simulink model "MSE491_Lab2_sample"  (R2018a)
settings: Solver=ode4  StartTime=0.0  StopTime=1  FixedStep=0.0002  MaxStep=1e-4  RelTol=1e-3  EnableMultiTasking=on
settings Model: Creator=jw  LastModifiedBy=jw
settings DataIOCC: LimitDataPoints=on  SaveFormat=Array  SignalLoggingSaveFormat=ModelDataLogs
settings OptimizationCC: InitFltsAndDblsToZero=on  LifeSpan=inf
settings DebuggingCC: SaveWithParameterizedLinksMsg=none  UnderspecifiedInitializationDetection=Classic  MergeDetectMultiDrivingBlocksExec=none  SignalResolutionControl=TryResolveAllWithWarning  SolverPrmCheckMsg=warning  MultiTaskDSMMsg=warning  MultiTaskCondExecSysMsg=none  FcnCallInpInsideContextMsg=warning  SFUnexpectedBacktrackingDiag=warning  SFNoUnconditionalDefaultTransitionDiag=warning  SFExecutionAtInitializationDiag=none
settings HardwareCC: ProdBitPerPointer=32  ProdBitPerSizeT=32  ProdBitPerPtrDiffT=32  ProdLargestAtomicFloat=None  ProdIntDivRoundTo=Undefined  ProdEndianess=Unspecified  ProdWordSize=32  ProdHWDeviceType=32-bit Generic
settings ModelReferenceCC: PropagateSignalLabelsOutOfModel=off
settings CodeAppCC: StateflowObjectComments=on
settings GRTTargetCC: TargetFcnLib=ansi_tfl_tmw.mat  TargetLangStandard=C89/C90 (ANSI)  CombineOutputUpdateFcns=off  GRTInterface=on
settings ConfigComp: CovMetricSettings=dw  CovHtmlReporting=on  CovSaveCumulativeToWorkspaceVar=on  CovSaveSingleToWorkspaceVar=on  CovExternalEMLEnable=off

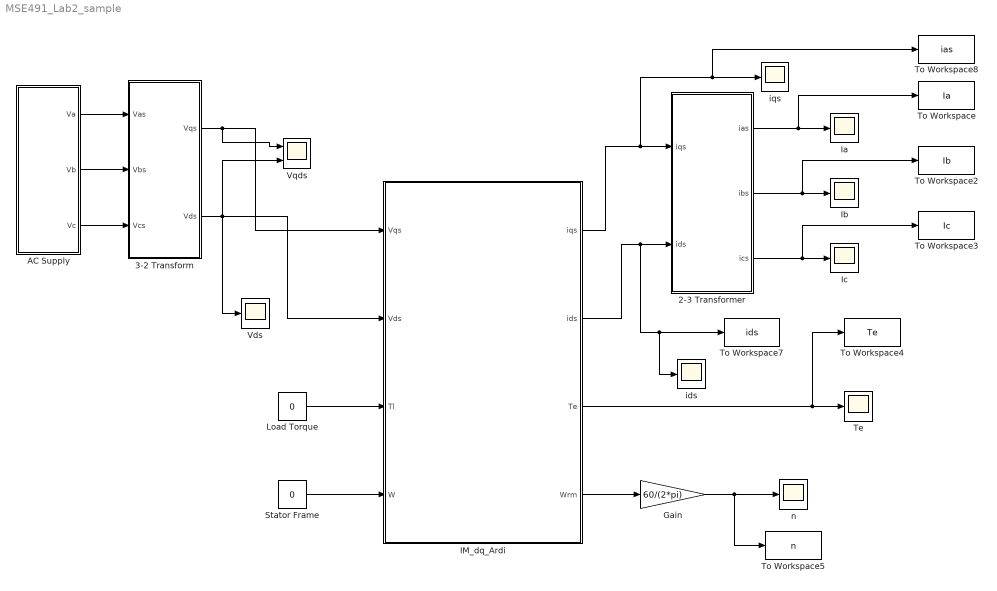
== system MSE491_Lab2_sample ==
  2-3 Transformer : Subsystem
  3-2 Transform : Subsystem
  AC Supply : Subsystem  Description=g
  Gain : Gain  Gain=60/(2*pi)
  IM_dq_Ardi : Subsystem
  Ia : Scope
  Ib : Scope
  Ic : Scope
  Load Torque : Constant  Value=0
  Stator Frame : Constant  Value=0
  Te : Scope
  To Workspace : ToWorkspace  VariableName=Ia  SampleTime=-1
  To Workspace2 : ToWorkspace  VariableName=Ib  SampleTime=-1
  To Workspace3 : ToWorkspace  VariableName=Ic  SampleTime=-1
  To Workspace4 : ToWorkspace  VariableName=Te  SampleTime=-1
  To Workspace5 : ToWorkspace  VariableName=n  SampleTime=-1
  To Workspace7 : ToWorkspace  VariableName=ids  SampleTime=-1
  To Workspace8 : ToWorkspace  VariableName=ias  SampleTime=-1
  Vds : Scope
  Vqds : Scope  NumInputPorts=2
  ids : Scope
  iqs : Scope
  n : Scope
  wires:
  AC Supply/1(Va) -> 3-2 Transform/1(Vas)
  AC Supply/2(Vb) -> 3-2 Transform/2(Vbs)
  AC Supply/3(Vc) -> 3-2 Transform/3(Vcs)
  3-2 Transform/1(Vqs) -> Vqds/1, IM_dq_Ardi/1(Vqs)
  3-2 Transform/2(Vds) -> Vds/1, Vqds/2, IM_dq_Ardi/2(Vds)
  2-3 Transformer/1(ias) -> Ia/1, To Workspace/1
  2-3 Transformer/2(ibs) -> Ib/1, To Workspace2/1
  2-3 Transformer/3(ics) -> Ic/1, To Workspace3/1
  Load Torque/1 -> IM_dq_Ardi/3(Tl)
  Stator Frame/1 -> IM_dq_Ardi/4(W)
  IM_dq_Ardi/1(iqs) -> 2-3 Transformer/1(iqs), iqs/1, To Workspace8/1
  IM_dq_Ardi/2(ids) -> 2-3 Transformer/2(ids), ids/1, To Workspace7/1
  IM_dq_Ardi/4(Wrm) -> Gain/1
  Gain/1 -> n/1, To Workspace5/1
  IM_dq_Ardi/3(Te) -> Te/1, To Workspace4/1

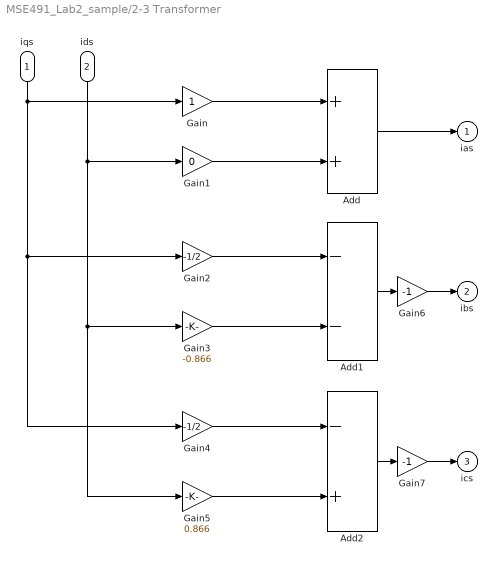
== system MSE491_Lab2_sample/2-3 Transformer ==
  iqs : Inport
  ids : Inport  Port=2
  Add : Sum
  Add1 : Sum  Inputs=--
  Add2 : Sum  Inputs=-+
  Gain : Gain
  Gain1 : Gain  Gain=0
  Gain2 : Gain  Gain=-1/2
  Gain3 : Gain  Gain=-0.866
  Gain4 : Gain  Gain=-1/2
  Gain5 : Gain  Gain=0.866
  Gain6 : Gain  Gain=-1
  Gain7 : Gain  Gain=-1
  ias : Outport  InitialOutput=0
  ibs : Outport  Port=2  InitialOutput=0
  ics : Outport  Port=3  InitialOutput=0
  wires:
  Gain/1 -> Add/1
  Gain1/1 -> Add/2
  Gain2/1 -> Add1/1
  Gain3/1 -> Add1/2
  Gain4/1 -> Add2/1
  Gain5/1 -> Add2/2
  Add2/1 -> Gain7/1
  Add1/1 -> Gain6/1
  Add/1 -> ias/1
  iqs/1 -> Gain/1, Gain2/1, Gain4/1
  ids/1 -> Gain1/1, Gain3/1, Gain5/1
  Gain6/1 -> ibs/1
  Gain7/1 -> ics/1

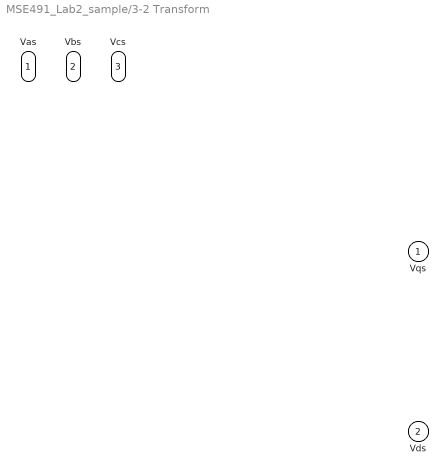
== system MSE491_Lab2_sample/3-2 Transform ==
  Vas : Inport
  Vbs : Inport  Port=2
  Vcs : Inport  Port=3
  Vqs : Outport  InitialOutput=0
  Vds : Outport  Port=2  InitialOutput=0

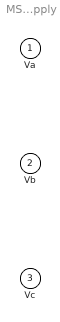
== system MSE491_Lab2_sample/AC Supply ==
  Va : Outport  InitialOutput=0
  Vb : Outport  Port=2  InitialOutput=0
  Vc : Outport  Port=3  InitialOutput=0

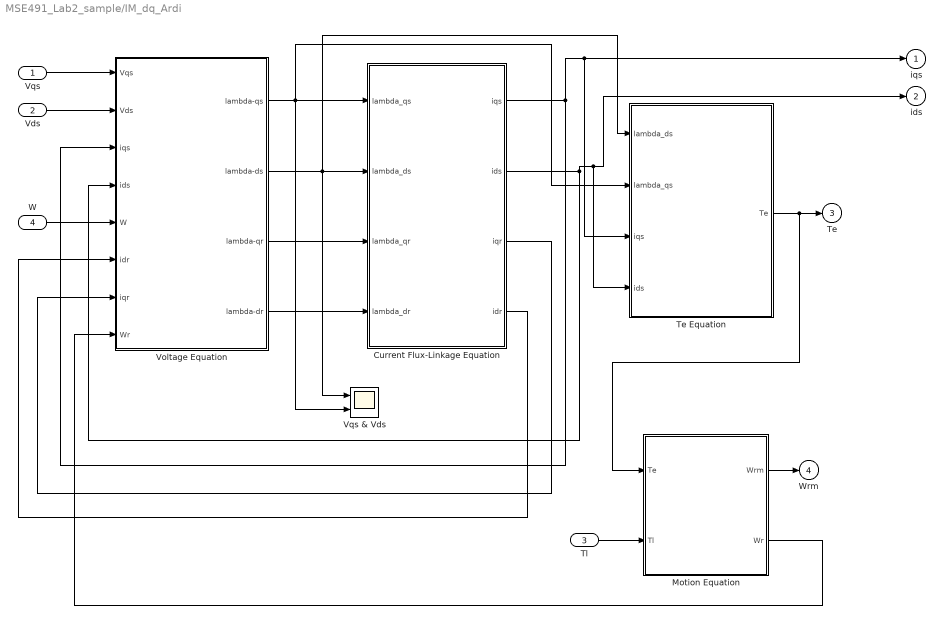
== system MSE491_Lab2_sample/IM_dq_Ardi ==
  Vqs : Inport
  Vds : Inport  Port=2
  Tl : Inport  Port=3
  W : Inport  Port=4
  Current Flux-Linkage Equation : Subsystem
  Motion Equation : Subsystem
  Te Equation : Subsystem
  Voltage Equation : Subsystem
  Vqs & Vds : Scope  NumInputPorts=2
  iqs : Outport  InitialOutput=0
  ids : Outport  Port=2  InitialOutput=0
  Te : Outport  Port=3  InitialOutput=0
  Wrm : Outport  Port=4  InitialOutput=0
  wires:
  Vqs/1 -> Voltage Equation/1(Vqs)
  Vds/1 -> Voltage Equation/2(Vds)
  Tl/1 -> Motion Equation/2(Tl)
  W/1 -> Voltage Equation/5(W)
  Te Equation/1(Te) -> Te/1, Motion Equation/1(Te)
  Current Flux-Linkage Equation/1(iqs) -> Voltage Equation/3(iqs), iqs/1, Te Equation/3(iqs)
  Current Flux-Linkage Equation/2(ids) -> Voltage Equation/4(ids), ids/1, Te Equation/4(ids)
  Current Flux-Linkage Equation/3(iqr) -> Voltage Equation/7(iqr)
  Voltage Equation/1(lambda-qs) -> Vqs & Vds/2, Current Flux-Linkage Equation/1(lambda_qs), Te Equation/2(lambda_qs)
  Voltage Equation/2(lambda-ds) -> Te Equation/1(lambda_ds), Vqs & Vds/1, Current Flux-Linkage Equation/2(lambda_ds)
  Voltage Equation/3(lambda-qr) -> Current Flux-Linkage Equation/3(lambda_qr)
  Voltage Equation/4(lambda-dr) -> Current Flux-Linkage Equation/4(lambda_dr)
  Current Flux-Linkage Equation/4(idr) -> Voltage Equation/6(idr)
  Motion Equation/2(Wr) -> Voltage Equation/8(Wr)
  Motion Equation/1(Wrm) -> Wrm/1

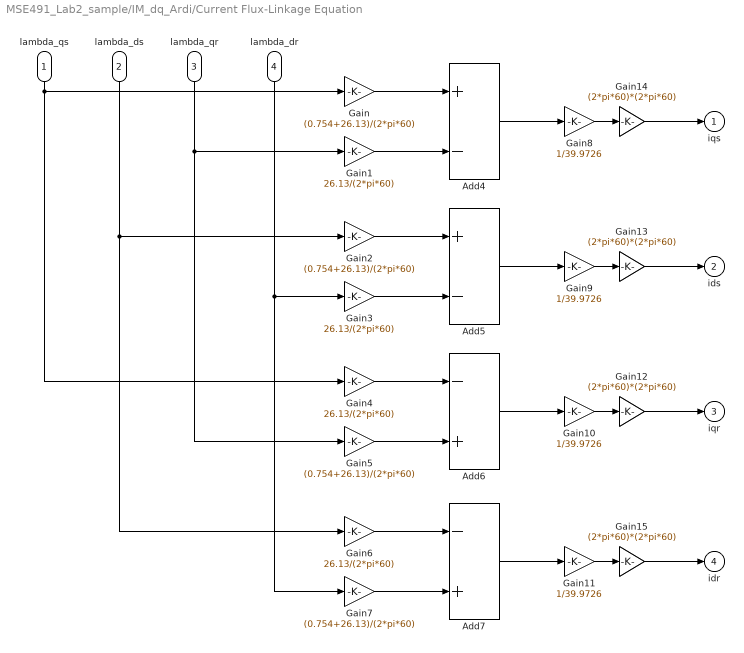
== system MSE491_Lab2_sample/IM_dq_Ardi/Current Flux-Linkage Equation ==
  lambda_qs : Inport
  lambda_ds : Inport  Port=2
  lambda_qr : Inport  Port=3
  lambda_dr : Inport  Port=4
  Add4 : Sum  Inputs=+-
  Add5 : Sum  Inputs=+-
  Add6 : Sum  Inputs=-+
  Add7 : Sum  Inputs=-+
  Gain{,2,5,7} (4 alike) : Gain  Gain=(0.754+26.13)/(2*pi*60)
  Gain{1,3..4,6} (4 alike) : Gain  Gain=26.13/(2*pi*60)
  Gain{8..11} (4 alike) : Gain  Gain=1/39.9726
  Gain{12..15} (4 alike) : Gain  Gain=(2*pi*60)*(2*pi*60)
  iqs : Outport  InitialOutput=0
  ids : Outport  Port=2  InitialOutput=0
  iqr : Outport  Port=3  InitialOutput=0
  idr : Outport  Port=4  InitialOutput=0
  wires:
  Gain1/1 -> Add4/2
  Gain/1 -> Add4/1
  Gain2/1 -> Add5/1
  Gain3/1 -> Add5/2
  Gain4/1 -> Add6/1
  Gain5/1 -> Add6/2
  Gain6/1 -> Add7/1
  Gain7/1 -> Add7/2
  Add4/1 -> Gain8/1
  Add5/1 -> Gain9/1
  Add6/1 -> Gain10/1
  Add7/1 -> Gain11/1
  lambda_qs/1 -> Gain/1, Gain4/1
  lambda_qr/1 -> Gain1/1, Gain5/1
  Gain10/1 -> Gain12/1
  Gain9/1 -> Gain13/1
  Gain8/1 -> Gain14/1
  Gain11/1 -> Gain15/1
  lambda_ds/1 -> Gain2/1, Gain6/1
  lambda_dr/1 -> Gain3/1, Gain7/1
  Gain14/1 -> iqs/1
  Gain13/1 -> ids/1
  Gain12/1 -> iqr/1
  Gain15/1 -> idr/1

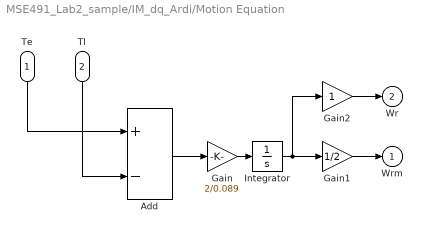
== system MSE491_Lab2_sample/IM_dq_Ardi/Motion Equation ==
  Te : Inport
  Tl : Inport  Port=2
  Add : Sum  Inputs=+-
  Gain : Gain  Gain=2/0.089
  Gain1 : Gain  Gain=1/2
  Gain2 : Gain
  Integrator : Integrator
  Wrm : Outport  InitialOutput=0
  Wr : Outport  Port=2  InitialOutput=0
  wires:
  Te/1 -> Add/1
  Tl/1 -> Add/2
  Gain/1 -> Integrator/1
  Add/1 -> Gain/1
  Integrator/1 -> Gain2/1, Gain1/1
  Gain2/1 -> Wr/1
  Gain1/1 -> Wrm/1

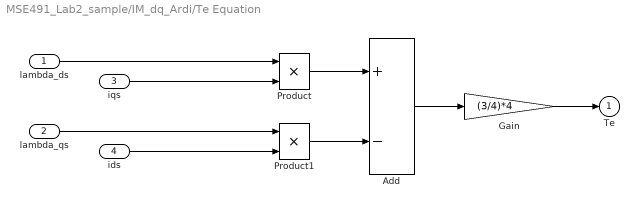
== system MSE491_Lab2_sample/IM_dq_Ardi/Te Equation ==
  lambda_ds : Inport
  lambda_qs : Inport  Port=2
  iqs : Inport  Port=3
  ids : Inport  Port=4
  Add : Sum  Inputs=+-
  Gain : Gain  Gain=(3/4)*4
  Product : Product  RndMeth=Zero
  Product1 : Product  RndMeth=Zero
  Te : Outport  InitialOutput=0
  wires:
  Gain/1 -> Te/1
  Add/1 -> Gain/1
  lambda_ds/1 -> Product/1
  iqs/1 -> Product/2
  lambda_qs/1 -> Product1/1
  ids/1 -> Product1/2
  Product/1 -> Add/1
  Product1/1 -> Add/2

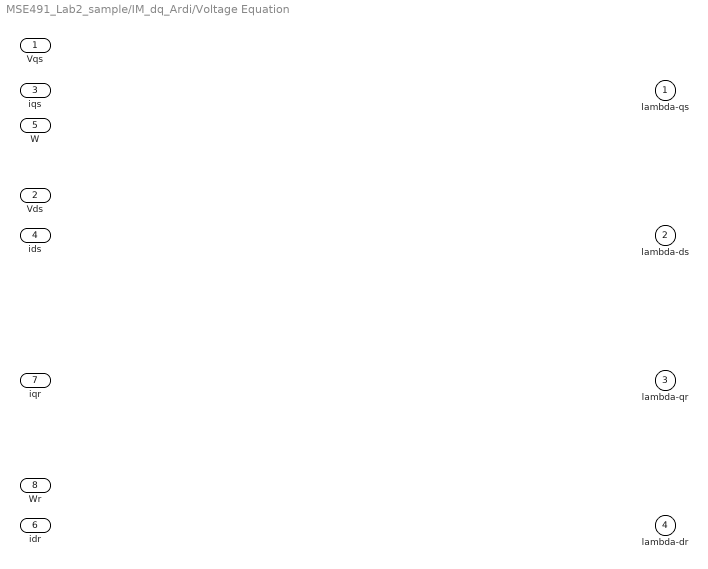
== system MSE491_Lab2_sample/IM_dq_Ardi/Voltage Equation ==
  Vqs : Inport
  Vds : Inport  Port=2
  iqs : Inport  Port=3
  ids : Inport  Port=4
  W : Inport  Port=5
  idr : Inport  Port=6
  iqr : Inport  Port=7
  Wr : Inport  Port=8
  lambda-qs : Outport  InitialOutput=0
  lambda-ds : Outport  Port=2  InitialOutput=0
  lambda-qr : Outport  Port=3  InitialOutput=0
  lambda-dr : Outport  Port=4  InitialOutput=0
